simulink model "main"  (R2022a)
settings: Solver=FixedStepDiscrete  StartTime=0.0  StopTime=Inf  FixedStep=(50e-6)-(sim_en*4.995e-5)  RelTol=1e-3  EnableMultiTasking=on
model workspace (MAT data in the model file):
  Param : Simulink.Parameter (value not decoded)
  ac_ok : Simulink.Signal (value not decoded)
  ac_ok_120 : Simulink.Signal (value not decoded)
  bulk_voltage : Simulink.Signal (value not decoded)
  burstduty_integ_max : Simulink.Signal (value not decoded)
  burstduty_integ_min : Simulink.Signal (value not decoded)
  burstduty_ki : Simulink.Signal (value not decoded)
  burstduty_kp : Simulink.Signal (value not decoded)
  calib_ok : Simulink.Signal (value not decoded)
  can_addr1 : Simulink.Signal (value not decoded)
  can_addr2 : Simulink.Signal (value not decoded)
  can_addr3 : Simulink.Signal (value not decoded)
  can_addr4 : Simulink.Signal (value not decoded)
  can_data_rx : Simulink.Signal (value not decoded)
  can_data_tx : Simulink.Signal (value not decoded)
  can_timeout_120 : Simulink.Signal (value not decoded)
  chksum_scircv : Simulink.Signal (value not decoded)
  clllc_en_120 : Simulink.Signal (value not decoded)
  clllc_fault_120 : Simulink.Signal (value not decoded)
  clllc_ok_120 : Simulink.Signal (value not decoded)
  cmpss1h : Simulink.Signal (value not decoded)
  cmpss1l : Simulink.Signal (value not decoded)
  cmpss2h : Simulink.Signal (value not decoded)
  cmpss2l : Simulink.Signal (value not decoded)
  cmpss3h : Simulink.Signal (value not decoded)
  cmpss3l : Simulink.Signal (value not decoded)
  cmpss4h : Simulink.Signal (value not decoded)
  cmpss4l : Simulink.Signal (value not decoded)
  cmpss5h : Simulink.Signal (value not decoded)
  cmpss5l : Simulink.Signal (value not decoded)
  cmpss6h : Simulink.Signal (value not decoded)
  cmpss6l : Simulink.Signal (value not decoded)
  cmpss7h : Simulink.Signal (value not decoded)
  cmpss7l : Simulink.Signal (value not decoded)
  cmpss8h : Simulink.Signal (value not decoded)
  cmpss8l : Simulink.Signal (value not decoded)
  cnt_idle : Simulink.Signal (value not decoded)
  cnt_orps : Simulink.Signal (value not decoded)
  cnt_scircv : Simulink.Signal (value not decoded)
  cnt_scixmt : Simulink.Signal (value not decoded)
  cnt_scixmt_func : Simulink.Signal (value not decoded)
  cnt_temp_mux : Simulink.Signal (value not decoded)
  cnt_vdroop : Simulink.Signal (value not decoded)
  config_ok : Simulink.Signal (value not decoded)
  control_en : Simulink.Signal (value not decoded)
  cp_ready_120 : Simulink.Signal (value not decoded)
  d2d_en : Simulink.Signal (value not decoded)
  dchg_off : Simulink.Signal (value not decoded)
  debug_dacb : Simulink.Signal (value not decoded)
  debug_dacc : Simulink.Signal (value not decoded)
  debug_msg1 : Simulink.Signal (value not decoded)
  debug_msg2 : Simulink.Signal (value not decoded)
  debug_msg3 : Simulink.Signal (value not decoded)
  debug_msg4 : Simulink.Signal (value not decoded)
  debug_msg5 : Simulink.Signal (value not decoded)
  debug_msg6 : Simulink.Signal (value not decoded)
  dir_v2g : Simulink.Signal (value not decoded)
  eoss_llc1 : Simulink.Signal (value not decoded)
  eoss_llc2 : Simulink.Signal (value not decoded)
  eoss_orps : Simulink.Signal (value not decoded)
  fault_ocp : Simulink.Signal (value not decoded)
  fault_otp : Simulink.Signal (value not decoded)
  fault_ovp : Simulink.Signal (value not decoded)
  fut_en : Simulink.Signal (value not decoded)
  fwd_en_120 : Simulink.Signal (value not decoded)
  gain_llc1_sec_idc : Simulink.Signal (value not decoded)
  gain_llc1_temp_sr : Simulink.Signal (value not decoded)
  gain_llc2_sec_idc : Simulink.Signal (value not decoded)
  gain_vbat : Simulink.Signal (value not decoded)
  gain_vbulk : Simulink.Signal (value not decoded)
  gain_vout : Simulink.Signal (value not decoded)
  input_current_phasea : Simulink.Signal (value not decoded)
  input_current_phaseb : Simulink.Signal (value not decoded)
  input_current_phasec : Simulink.Signal (value not decoded)
  input_freq : Simulink.Signal (value not decoded)
  input_power : Simulink.Signal (value not decoded)
  input_voltage_phasea : Simulink.Signal (value not decoded)
  input_voltage_phaseb : Simulink.Signal (value not decoded)
  input_voltage_phasec : Simulink.Signal (value not decoded)
  ishare_arbiter : Simulink.Signal (value not decoded)
  ishare_thresh : Simulink.Signal (value not decoded)
  led_g : Simulink.Signal (value not decoded)
  led_r : Simulink.Signal (value not decoded)
  led_y : Simulink.Signal (value not decoded)
  llc1_burst_integ : Simulink.Signal (value not decoded)
  llc1_burstduty_buffer : Simulink.Signal (value not decoded)
  llc1_pfm_error : Simulink.Signal (value not decoded)
  llc1_pfm_integ : Simulink.Signal (value not decoded)
  llc1_pfm_prop : Simulink.Signal (value not decoded)
  llc1_pri_idc : Simulink.Signal (value not decoded)
  llc1_ps_buffer : Simulink.Signal (value not decoded)
  llc1_pspwm_error : Simulink.Signal (value not decoded)
  llc1_pspwm_integ : Simulink.Signal (value not decoded)
  llc1_pspwm_prop : Simulink.Signal (value not decoded)
  llc1_sec_idc : Simulink.Signal (value not decoded)
  llc1_temp_sr : Simulink.Signal (value not decoded)
  llc1_ts_tbctr_buffer : Simulink.Signal (value not decoded)
  llc2_burst_integ : Simulink.Signal (value not decoded)
  llc2_burstduty_buffer : Simulink.Signal (value not decoded)
  llc2_en : Simulink.Signal (value not decoded)
  llc2_en_buffer : Simulink.Signal (value not decoded)
  llc2_pfm_error : Simulink.Signal (value not decoded)
  llc2_pfm_integ : Simulink.Signal (value not decoded)
  llc2_pfm_prop : Simulink.Signal (value not decoded)
  llc2_pri_idc : Simulink.Signal (value not decoded)
  llc2_ps_buffer : Simulink.Signal (value not decoded)
  llc2_pspwm_error : Simulink.Signal (value not decoded)
  llc2_pspwm_integ : Simulink.Signal (value not decoded)
  llc2_pspwm_prop : Simulink.Signal (value not decoded)
  llc2_sec_idc : Simulink.Signal (value not decoded)
  llc2_temp_sr : Simulink.Signal (value not decoded)
  llc2_ts_tbctr_buffer : Simulink.Signal (value not decoded)
  loop_adcint : Simulink.Signal (value not decoded)
  loop_control : Simulink.Signal (value not decoded)
  loop_idle : Simulink.Signal (value not decoded)
  mid_bulk_voltage : Simulink.Signal (value not decoded)
  mode_120 : Simulink.Signal (value not decoded)
  mode_cc_cv : Simulink.Signal (value not decoded)
  myParam : mpt.Parameter (value not decoded)
  obc_ok_120 : Simulink.Signal (value not decoded)
  offset_llc1_sec_idc : Simulink.Signal (value not decoded)
  offset_llc1_temp_sr : Simulink.Signal (value not decoded)
  offset_llc2_sec_idc : Simulink.Signal (value not decoded)
  offset_vbat : Simulink.Signal (value not decoded)
  offset_vbulk : Simulink.Signal (value not decoded)
  offset_vout : Simulink.Signal (value not decoded)
  openloop_en : Simulink.Signal (value not decoded)
  openloop_fault_en : Simulink.Signal (value not decoded)
  ot_fault_120 : Simulink.Signal (value not decoded)
  pfc_en : Simulink.Signal (value not decoded)
  pfc_en_120 : Simulink.Signal (value not decoded)
  pfc_fw_revision : Simulink.Signal (value not decoded)
  pfc_fw_revision_bootloader : Simulink.Signal (value not decoded)
  pfc_fw_revision_debug : Simulink.Signal (value not decoded)
  pfc_ok : Simulink.Signal (value not decoded)
  pfc_ok_120 : Simulink.Signal (value not decoded)
  pfm_a0 : Simulink.Signal (value not decoded)
  pfm_a1 : Simulink.Signal (value not decoded)
  pfm_integ_max : Simulink.Signal (value not decoded)
  pfm_integ_min : Simulink.Signal (value not decoded)
  pfm_ki : Simulink.Signal (value not decoded)
  pfm_kp : Simulink.Signal (value not decoded)
  pri_fut_en : Simulink.Signal (value not decoded)
  pri_fut_en_buffer : Simulink.Signal (value not decoded)
  pri_halfbridge_en : Simulink.Signal (value not decoded)
  pri_halfbridge_en_buffer : Simulink.Signal (value not decoded)
  pspwm_integ_max : Simulink.Signal (value not decoded)
  pspwm_integ_min : Simulink.Signal (value not decoded)
  pspwm_ki : Simulink.Signal (value not decoded)
  pspwm_kp : Simulink.Signal (value not decoded)
  ref_idclink_max : Simulink.Signal (value not decoded)
  ref_iout : Simulink.Signal (value not decoded)
  ref_iout_calib : Simulink.Signal (value not decoded)
  ref_iout_llc1 : Simulink.Signal (value not decoded)
  ref_iout_llc1_calib : Simulink.Signal (value not decoded)
  ref_iout_llc2 : Simulink.Signal (value not decoded)
  ref_iout_llc2_calib : Simulink.Signal (value not decoded)
  ref_pout : Simulink.Signal (value not decoded)
  ref_ss_llc1 : Simulink.Signal (value not decoded)
  ref_ss_llc2 : Simulink.Signal (value not decoded)
  ref_ss_orps : Simulink.Signal (value not decoded)
  ref_vbat : Simulink.Signal (value not decoded)
  ref_vbat_calib : Simulink.Signal (value not decoded)
  ref_vbulk : Simulink.Signal (value not decoded)
  ref_vbulk_calib : Simulink.Signal (value not decoded)
  ref_vbulk_llc1_calib : Simulink.Signal (value not decoded)
  ref_vbulk_llc2_calib : Simulink.Signal (value not decoded)
  ref_vout : Simulink.Signal (value not decoded)
  ref_vout_calib : Simulink.Signal (value not decoded)
  relay_en : Simulink.Signal (value not decoded)
  reset_flag : Simulink.Signal (value not decoded)
  rev_en_120 : Simulink.Signal (value not decoded)
  runtime_control : Simulink.Signal (value not decoded)
  runtime_idle : Simulink.Signal (value not decoded)
  scircv_buffer : Simulink.Signal (value not decoded)
  scircv_buffer_tmp : Simulink.Signal (value not decoded)
  scircv_buffer_tmp_idx0 : Simulink.Signal (value not decoded)
  scircv_chksum : Simulink.Signal (value not decoded)
  scircv_chksum_ok : Simulink.Signal (value not decoded)
  scircv_parse_ok : Simulink.Signal (value not decoded)
  scixmt_buffer : Simulink.Signal (value not decoded)
  scixmt_chksum : Simulink.Signal (value not decoded)
  scixmt_func : Simulink.Signal (value not decoded)
  scixmt_word0_lsb : Simulink.Signal (value not decoded)
  scixmt_word0_msb : Simulink.Signal (value not decoded)
  scixmt_word1_lsb : Simulink.Signal (value not decoded)
  scixmt_word1_msb : Simulink.Signal (value not decoded)
  scixmt_word2_lsb : Simulink.Signal (value not decoded)
  scixmt_word2_msb : Simulink.Signal (value not decoded)
  scixmt_wr : Simulink.Signal (value not decoded)
  ss_step : Simulink.Signal (value not decoded)
  state_calib : Simulink.Signal (value not decoded)
  state_control : Simulink.Signal (value not decoded)
  state_hkeep : Simulink.Signal (value not decoded)
  status_cmpss : Simulink.Signal (value not decoded)
  status_control : Simulink.Signal (value not decoded)
  status_digin : Simulink.Signal (value not decoded)
  status_digout : Simulink.Signal (value not decoded)
  status_fault : Simulink.Signal (value not decoded)
  status_input : Simulink.Signal (value not decoded)
  status_pfc : Simulink.Signal (value not decoded)
  temp_inlet : Simulink.Signal (value not decoded)
  temp_llc1_fet_hs : Simulink.Signal (value not decoded)
  temp_llc2_fet_hs : Simulink.Signal (value not decoded)
  temp_mux : Simulink.Signal (value not decoded)
  temp_mux_s0 : Simulink.Signal (value not decoded)
  temp_mux_s1 : Simulink.Signal (value not decoded)
  temp_mux_s2 : Simulink.Signal (value not decoded)
  temp_outlet : Simulink.Signal (value not decoded)
  temp_pfc_fet_hsa : Simulink.Signal (value not decoded)
  temp_pfc_fet_hsb : Simulink.Signal (value not decoded)
  temp_pfc_fet_hsc : Simulink.Signal (value not decoded)
  temp_pfc_fet_lsa : Simulink.Signal (value not decoded)
  temp_pfc_fet_lsb : Simulink.Signal (value not decoded)
  temp_pfc_fet_lsc : Simulink.Signal (value not decoded)
  test_mode : Simulink.Signal (value not decoded)
  tfcv_cc : Simulink.Signal (value not decoded)
  tfcv_cc_llc2 : Simulink.Signal (value not decoded)
  tfcv_cv : Simulink.Signal (value not decoded)
  tfcv_sr_en : Simulink.Signal (value not decoded)
  tfv_assert_llc1_pri_idc : Simulink.Signal (value not decoded)
  tfv_assert_llc1_sec_idc : Simulink.Signal (value not decoded)
  tfv_assert_llc1_temp_sr : Simulink.Signal (value not decoded)
  tfv_assert_llc2_pri_idc : Simulink.Signal (value not decoded)
  tfv_assert_llc2_sec_idc : Simulink.Signal (value not decoded)
  tfv_assert_llc2_temp_sr : Simulink.Signal (value not decoded)
  tfv_assert_temp_outlet : Simulink.Signal (value not decoded)
  tfv_assert_vaux_uv : Simulink.Signal (value not decoded)
  tfv_assert_vbat : Simulink.Signal (value not decoded)
  tfv_assert_vbulk : Simulink.Signal (value not decoded)
  tfv_assert_vout : Simulink.Signal (value not decoded)
  tfv_cnt_tz : Simulink.Signal (value not decoded)
  tfv_deassert_llc1_pri_idc : Simulink.Signal (value not decoded)
  tfv_deassert_llc1_sec_idc : Simulink.Signal (value not decoded)
  tfv_deassert_llc1_temp_sr : Simulink.Signal (value not decoded)
  tfv_deassert_llc2_pri_idc : Simulink.Signal (value not decoded)
  tfv_deassert_llc2_sec_idc : Simulink.Signal (value not decoded)
  tfv_deassert_llc2_temp_sr : Simulink.Signal (value not decoded)
  tfv_deassert_temp_outlet : Simulink.Signal (value not decoded)
  tfv_deassert_vaux_uv : Simulink.Signal (value not decoded)
  tfv_deassert_vbat : Simulink.Signal (value not decoded)
  tfv_deassert_vbulk : Simulink.Signal (value not decoded)
  tfv_deassert_vout : Simulink.Signal (value not decoded)
  tfv_llc1_pri_idc : Simulink.Signal (value not decoded)
  tfv_llc1_sec_idc : Simulink.Signal (value not decoded)
  tfv_llc1_temp_sr : Simulink.Signal (value not decoded)
  tfv_llc2_pri_idc : Simulink.Signal (value not decoded)
  tfv_llc2_sec_idc : Simulink.Signal (value not decoded)
  tfv_llc2_temp_sr : Simulink.Signal (value not decoded)
  tfv_temp_outlet : Simulink.Signal (value not decoded)
  tfv_vaux_uv : Simulink.Signal (value not decoded)
  tfv_vbat : Simulink.Signal (value not decoded)
  tfv_vbulk : Simulink.Signal (value not decoded)
  tfv_vout : Simulink.Signal (value not decoded)
  timer_1ms : Simulink.Signal (value not decoded)
  tz : Simulink.Signal (value not decoded)
  valve_en : Simulink.Signal (value not decoded)
  vaux : Simulink.Signal (value not decoded)
  vbat : Simulink.Signal (value not decoded)
  vbulk : Simulink.Signal (value not decoded)
  vout : Simulink.Signal (value not decoded)
undefined symbols (not defined in the file or in its folder): CAN_O_INT, CANA_BASE, Down, GPTRIP1SEL, GPTRIP2SEL, TZ1, TZ2, Up
libraries: hdlsllib x159, simulink x94, c2802xlib x32, c2837xDlib x19, c2807xlib x16, c280xlib x13, canmsglib x8, idelinklib_common x2, c2000lib x1, c281xlib x1
(part 8 of 20)

== system main/Task_Manager/Tmr_1mS/codegen ==
  Task_1mS : Subsystem  TreatAsAtomicUnit=on  ScheduleAs=Periodic partition  PartitionName=Task1mS  SystemSampleTime=1e-3
      settings: RTWFcnNameOpts=Use subsystem name  RTWFileNameOpts=Use subsystem name

== system main/Task_Manager/Tmr_1mS/sim ==

== system main/Task_Manager/Tmr_1s/codegen ==
  Task_1S : Subsystem  TreatAsAtomicUnit=on  ScheduleAs=Periodic partition  PartitionName=Task1S  SystemSampleTime=1
      settings: RTWFcnNameOpts=Use subsystem name  RTWFileNameOpts=Use subsystem name

== system main/Task_Manager/Tmr_1s/sim ==

== system main/Task_Manager/Tmr_20mS/codegen ==
  Task_20mS : Subsystem  TreatAsAtomicUnit=on  ScheduleAs=Periodic partition  PartitionName=Task20mS  SystemSampleTime=19e-3
      settings: RTWFcnNameOpts=Use subsystem name  RTWFileNameOpts=Use subsystem name

== system main/Task_Manager/Tmr_20mS/sim ==

== system main/Task_Manager/idle/cnt_idle ==
  function : TriggerPort  TriggerType=function-call  VariantControl=Variant
  Data Store Read : DataStoreRead  DataStoreName=cnt_idle  IndexOptions=Index vector (dialog)  Indices=1  OutputSizes=1
  If : If  IfExpression=u1 < 5
  cnt_idle : Subsystem  TreatAsAtomicUnit=on
  cnt_idle_sat : Subsystem  TreatAsAtomicUnit=on
  wires:
  Data Store Read/1 -> If/1
  If/1 -> cnt_idle/Action
  If/2 -> cnt_idle_sat/Action

== system main/Task_Manager/idle/idle_task ==
  sim_digin : Inport
  function : TriggerPort  TriggerType=function-call  VariantControl=Variant
  Data Store Read : DataStoreRead  DataStoreName=cnt_idle  IndexOptions=Index vector (dialog)  Indices=1  OutputSizes=1
  Switch Case : SwitchCase  CaseConditions={0,1,2,3,4,5}
  calib : Subsystem  TreatAsAtomicUnit=on
  comm_npc : Subsystem  Commented=on  TreatAsAtomicUnit=on
  debug_dac : Subsystem  Commented=on  TreatAsAtomicUnit=on
  debug_uart1 : Subsystem  Commented=on  TreatAsAtomicUnit=on
  hkeep : Subsystem  TreatAsAtomicUnit=on
  status : Subsystem  TreatAsAtomicUnit=on
  uartx : Subsystem  Commented=on  TreatAsAtomicUnit=on
  watchdog : Subsystem  TreatAsAtomicUnit=on
  sim_digout : Outport
  wires:
  Switch Case/1 -> watchdog/Action
  Switch Case/3 -> hkeep/Action
  Switch Case/5 -> comm_npc/Action
  Switch Case/6 -> debug_dac/Action
  status/1(sim_digout) -> sim_digout/1
  Switch Case/4 -> status/Action
  Data Store Read/1 -> Switch Case/1
  Switch Case/2 -> calib/Action
  sim_digin/1 -> status/1(sim_digin)

== system main/Task_Manager/init/codegen ==
  init : Subsystem
      settings: RTWSystemCode=Inline  RTWFcnNameOpts=Use subsystem name  RTWFileNameOpts=Use subsystem name

== system main/Task_Manager/init/sim ==

== system main/interrupt_adca/burst_control/burst/disPulse ==
  f : TriggerPort  TriggerType=function-call  VariantControl=(inherit)
      settings: CopyFcn=Stateflow.SLINSF.SimulinkMan.removeBlockPreDeleteFcn  PreDeleteFcn=Stateflow.SLINSF.SimulinkMan.unsafePredeleteFcn
  Data Store Read1 : DataStoreRead  DataStoreName=dir_v2g  IndexOptions=Index vector (dialog)  Indices=1  OutputSizes=1
  Rate Transition : RateTransition  Deterministic=off
  Variant Subsystem : Subsystem  Variant=on
  wires:
  Data Store Read1/1 -> Rate Transition/1
  Rate Transition/1 -> Variant Subsystem/1(dir_v2g)

== system main/interrupt_adca/burst_control/burst/disPwm ==
  f : TriggerPort  TriggerType=function-call  VariantControl=(inherit)
      settings: CopyFcn=Stateflow.SLINSF.SimulinkMan.removeBlockPreDeleteFcn  PreDeleteFcn=Stateflow.SLINSF.SimulinkMan.unsafePredeleteFcn
  disPwm : Subsystem  Variant=on

== system main/interrupt_adca/burst_control/burst/enPulse ==
  f : TriggerPort  TriggerType=function-call  VariantControl=(inherit)
      settings: CopyFcn=Stateflow.SLINSF.SimulinkMan.removeBlockPreDeleteFcn  PreDeleteFcn=Stateflow.SLINSF.SimulinkMan.unsafePredeleteFcn
  enPwm : Subsystem  Variant=on

== system main/interrupt_adca/get_adc/adc_variant_subsystem ==
  note: 1) Add Subsystem or Model blocks as valid variant choices.
      | 2) You cannot connect blocks at this level. At simulation, connectivity is automatically
      | determined, based on the active variant and port name matching.
  note: ADCA:
      | llc1_sec_idc
      | llc1_pri_idc
      | vout
  note: ADCB :
      | vaux
      | vbulk
      | temp_mux
  sim_adca : Inport
  sim_adcb : Inport  Port=2
  codegen : Subsystem  VariantControl=sim_en==0
  sim : Subsystem  VariantControl=sim_en==1

== system main/interrupt_adca/to_simulated_plant/codegen ==
  signal_pwm_cllc1 : Outport

== system main/interrupt_adca/to_simulated_plant/sim ==
  Data Store Read3 : DataStoreRead  DataStoreName=llc1_ps  IndexOptions=Index vector (dialog)  Indices=1  OutputSizes=1
  Data Store Read4 : DataStoreRead  DataStoreName=llc1_ts_tbctr  IndexOptions=Index vector (dialog)  Indices=1  OutputSizes=1
  Mux2 : Mux  Inputs=2
  signal_pwm_cllc1 : Outport
  wires:
  Data Store Read4/1 -> Mux2/1
  Data Store Read3/1 -> Mux2/2
  Mux2/1 -> signal_pwm_cllc1/1

== system main/interrupt_canrx/canrx_variant_subsystem/codegen ==
  Function-Call Generator2 : simulink/Ports & Subsystems/Function-Call Generator  sample_time=-1  numberOfIterations=1  DisallowWideOutput=off
  can_rcv : Subsystem  TreatAsAtomicUnit=on
  wires:
  Function-Call Generator2/1 -> can_rcv/Trigger

== system main/interrupt_canrx/canrx_variant_subsystem/sim ==
  sim_canrx : Inport
  Data Store Write1 : DataStoreWrite  DataStoreName=f32BurstDuty1  IndexOptions=Index vector (dialog)  Indices=1  OutputSizes=1
  Data Store Write2 : DataStoreWrite  DataStoreName=f32PhaseShift1  IndexOptions=Index vector (dialog)  Indices=1  OutputSizes=1
  Data Store Write3 : DataStoreWrite  DataStoreName=u8OpenLoopEn1  IndexOptions=Index vector (dialog)  Indices=1  OutputSizes=1
  Data Store Write5 : DataStoreWrite  DataStoreName=f32FreqPeriod1  IndexOptions=Index vector (dialog)  Indices=1  OutputSizes=1
  Demux : Demux
  wires:
  sim_canrx/1 -> Demux/1
  Demux/2 -> Data Store Write5/1
  Demux/3 -> Data Store Write2/1
  Demux/4 -> Data Store Write1/1
  Demux/1 -> Data Store Write3/1

== system main/Control_State_Machine/control/configSr/configXbarEpwmtrip/codegen ==
  dir_v2g : Inport
  If : If  IfExpression=(u1==0)  ElseIfExpressions=(u1==1)  ShowElse=off
  g2v_prifullbridge : Subsystem  TreatAsAtomicUnit=on
  v2g_prifullbridge : Subsystem  TreatAsAtomicUnit=on
  wires:
  dir_v2g/1 -> If/1
  If/2 -> v2g_prifullbridge/Action
  If/1 -> g2v_prifullbridge/Action

== system main/Control_State_Machine/control/configSr/configXbarEpwmtrip/sim ==
  dir_v2g : Inport
  If : If  IfExpression=(u1==0)
  g2v_prifullbridge : Subsystem  TreatAsAtomicUnit=on
  v2g_prifullbridge : Subsystem  TreatAsAtomicUnit=on
  wires:
  If/2 -> v2g_prifullbridge/Action
  dir_v2g/1 -> If/1
  If/1 -> g2v_prifullbridge/Action

== system main/Control_State_Machine/control/disPwm/disPwm/codegen ==
  note: EPwm1Regs.AQCSFRC.bit.CSFA = 0b01; //force low
      | EPwm1Regs.AQCSFRC.bit.CSFB = 0b01; //force low
      | EPwm2Regs.AQCSFRC.bit.CSFA = 0b01; //force low
      | EPwm2Regs.AQCSFRC.bit.CSFB = 0b01; //force low
      |
      | EPwm7Regs.AQCSFRC.bit.CSFA = 0b01; //force low
      | EPwm7Regs.AQCSFRC.bit.CSFB = 0b01; //force low
      | EPwm8Regs.AQCSFRC.bit.CSFA = 0b01; //force low
      | EPwm8Regs.AQCSFRC.bit.CSFB = 0b01; //force low
  System Outputs1 : Subsystem  VariantControl=Choice  mask(System Outputs){ShowInLibBrowser=0}
      mask prompts: ShowInLibBrowser "Simulink:masks:CustCodeMaskParam1_MP"
      settings: CopyFcn=cccopyfcn(gcb)  OpenFcn=ccopenfcn('System Outputs Function')
      mask Help: eval('feval(''rtwprivate'',''rtwhelpview'',''rtw_sys_outputs_block'')');
      mask DialogControl ShowInLibBrowser Prompt: Mask Parameter 1:
      mask Display: disp('System\nOutputs');

== system main/Control_State_Machine/control/disPwm/disPwm/sim ==
  note: Note:
      | 0 - disable forced low
      | 1 - forced low
  Constant : Constant  OutDataTypeStr=boolean
  Data Store Write : DataStoreWrite  DataStoreName=epwm1_aqcsfrc_csfa  IndexOptions=Index vector (dialog)  Indices=1  OutputSizes=1
  Data Store Write1 : DataStoreWrite  DataStoreName=epwm1_aqcsfrc_csfb  IndexOptions=Index vector (dialog)  Indices=1  OutputSizes=1
  Data Store Write2 : DataStoreWrite  DataStoreName=epwm2_aqcsfrc_csfa  IndexOptions=Index vector (dialog)  Indices=1  OutputSizes=1
  Data Store Write3 : DataStoreWrite  DataStoreName=epwm2_aqcsfrc_csfb  IndexOptions=Index vector (dialog)  Indices=1  OutputSizes=1
  Data Store Write4 : DataStoreWrite  DataStoreName=epwm7_aqcsfrc_csfa  IndexOptions=Index vector (dialog)  Indices=1  OutputSizes=1
  Data Store Write5 : DataStoreWrite  DataStoreName=epwm7_aqcsfrc_csfb  IndexOptions=Index vector (dialog)  Indices=1  OutputSizes=1
  Data Store Write6 : DataStoreWrite  DataStoreName=epwm8_aqcsfrc_csfa  IndexOptions=Index vector (dialog)  Indices=1  OutputSizes=1
  Data Store Write7 : DataStoreWrite  DataStoreName=epwm8_aqcsfrc_csfb  IndexOptions=Index vector (dialog)  Indices=1  OutputSizes=1
  wires:
  Constant/1 -> Data Store Write7/1, Data Store Write6/1, Data Store Write5/1, Data Store Write4/1, Data Store Write3/1, Data Store Write2/1, Data Store Write1/1, Data Store Write/1

== system main/Control_State_Machine/control/enableSR/enPwm/codegen ==
  note: EPwm1Regs.AQCSFRC.bit.CSFA = 0b0; //force disabled
      | EPwm1Regs.AQCSFRC.bit.CSFB = 0b0; //force disabled
      | EPwm2Regs.AQCSFRC.bit.CSFA = 0b0; //force disabled
      | EPwm2Regs.AQCSFRC.bit.CSFB = 0b0; //force disabled
      |
      | //Enable sync  rec
      | //EPwm7Regs.AQCSFRC.bit.CSFA = 0b0; //force disabled
      | //EPwm7Regs.AQCSFRC.bit.CSFB = 0b0; //force disabled
      | //EPwm8Regs.AQCSFRC.bit.CSFA = 0b0; //force disabled
      | //EPwm8Regs.AQCSFRC.bit.CSFB = 0b0; //force disabled
      |
      | //Disable sync rec
      | EPwm7Regs.AQCSFRC.bit.CSFA = 0b1; //force low
      | EPwm7Regs.AQCSFRC.bit.CSFB = 0b1; //force low
      | EPwm8Regs.AQCSFRC.bit.CSFA = 0b1; //force low
      | EPwm8Regs.AQCSFRC.bit.CSFB = 0b1; //force low
  System Outputs : Subsystem  mask(System Outputs){ShowInLibBrowser=0}
      mask prompts: ShowInLibBrowser "Simulink:masks:CustCodeMaskParam1_MP"
      settings: CopyFcn=cccopyfcn(gcb)  OpenFcn=ccopenfcn('System Outputs Function')
      mask Help: eval('feval(''rtwprivate'',''rtwhelpview'',''rtw_sys_outputs_block'')');
      mask Display: disp('System\nOutputs');

== system main/Control_State_Machine/control/enableSR/enPwm/sim ==
  note: LLC1 SEC
  note: LLC1 PRI
  note: EPwm1Regs.AQCSFRC.bit.CSFA = 0b0; //force disabled
      | EPwm1Regs.AQCSFRC.bit.CSFB = 0b0; //force disabled
      | EPwm2Regs.AQCSFRC.bit.CSFA = 0b0; //force disabled
      | EPwm2Regs.AQCSFRC.bit.CSFB = 0b0; //force disabled
      | EPwm7Regs.AQCSFRC.bit.CSFA = 0b0; //force disabled
      | EPwm7Regs.AQCSFRC.bit.CSFB = 0b0; //force disabled
      | EPwm8Regs.AQCSFRC.bit.CSFA = 0b0; //force disabled
      | EPwm8Regs.AQCSFRC.bit.CSFB = 0b0; //force disabled
  Constant{,1..7} (8 alike) : Constant  Value=0  OutDataTypeStr=boolean
  Data Store Write : DataStoreWrite  DataStoreName=epwm1_aqcsfrc_csfa  IndexOptions=Index vector (dialog)  Indices=1  OutputSizes=1
  Data Store Write1 : DataStoreWrite  DataStoreName=epwm1_aqcsfrc_csfb  IndexOptions=Index vector (dialog)  Indices=1  OutputSizes=1
  Data Store Write2 : DataStoreWrite  DataStoreName=epwm7_aqcsfrc_csfa  IndexOptions=Index vector (dialog)  Indices=1  OutputSizes=1
  Data Store Write3 : DataStoreWrite  DataStoreName=epwm7_aqcsfrc_csfb  IndexOptions=Index vector (dialog)  Indices=1  OutputSizes=1
  Data Store Write4 : DataStoreWrite  DataStoreName=epwm2_aqcsfrc_csfa  IndexOptions=Index vector (dialog)  Indices=1  OutputSizes=1
  Data Store Write5 : DataStoreWrite  DataStoreName=epwm2_aqcsfrc_csfb  IndexOptions=Index vector (dialog)  Indices=1  OutputSizes=1
  Data Store Write6 : DataStoreWrite  DataStoreName=epwm8_aqcsfrc_csfa  IndexOptions=Index vector (dialog)  Indices=1  OutputSizes=1
  Data Store Write7 : DataStoreWrite  DataStoreName=epwm8_aqcsfrc_csfb  IndexOptions=Index vector (dialog)  Indices=1  OutputSizes=1
  wires:
  Constant/1 -> Data Store Write/1
  Constant1/1 -> Data Store Write1/1
  Constant4/1 -> Data Store Write4/1
  Constant5/1 -> Data Store Write5/1
  Constant7/1 -> Data Store Write7/1
  Constant6/1 -> Data Store Write6/1
  Constant3/1 -> Data Store Write3/1
  Constant2/1 -> Data Store Write2/1

== system main/Control_State_Machine/control/initG2vCcBurst/initG2vCcBurst/codegen ==
  Constant : Constant  Value=0.0025  OutDataTypeStr=single
  Constant1 : Constant  Value=0.00025  OutDataTypeStr=single
  Constant2 : Constant  Value=0  OutDataTypeStr=single
  Constant3 : Constant  Value=100  OutDataTypeStr=single
  Data Store Write : DataStoreWrite  DataStoreName=burstduty_kp  IndexOptions=Index vector (dialog)  Indices=1  OutputSizes=1
  Data Store Write1 : DataStoreWrite  DataStoreName=burstduty_ki  IndexOptions=Index vector (dialog)  Indices=1  OutputSizes=1
  Data Store Write2 : DataStoreWrite  DataStoreName=burstduty_integ_min  IndexOptions=Index vector (dialog)  Indices=1  OutputSizes=1
  Data Store Write3 : DataStoreWrite  DataStoreName=burstduty_integ_max  IndexOptions=Index vector (dialog)  Indices=1  OutputSizes=1
  wires:
  Constant3/1 -> Data Store Write3/1
  Constant2/1 -> Data Store Write2/1
  Constant1/1 -> Data Store Write1/1
  Constant/1 -> Data Store Write/1

== system main/Control_State_Machine/control/initG2vCcBurst/initG2vCcBurst/sim ==
  Constant : Constant  Value=40e-1  OutDataTypeStr=single
  Constant1 : Constant  Value=40e-2  OutDataTypeStr=single
  Constant2 : Constant  Value=0  OutDataTypeStr=single
  Constant3 : Constant  Value=100  OutDataTypeStr=single
  Data Store Write : DataStoreWrite  DataStoreName=burstduty_kp  IndexOptions=Index vector (dialog)  Indices=1  OutputSizes=1
  Data Store Write1 : DataStoreWrite  DataStoreName=burstduty_ki  IndexOptions=Index vector (dialog)  Indices=1  OutputSizes=1
  Data Store Write2 : DataStoreWrite  DataStoreName=burstduty_integ_min  IndexOptions=Index vector (dialog)  Indices=1  OutputSizes=1
  Data Store Write3 : DataStoreWrite  DataStoreName=burstduty_integ_max  IndexOptions=Index vector (dialog)  Indices=1  OutputSizes=1
  wires:
  Constant2/1 -> Data Store Write2/1
  Constant3/1 -> Data Store Write3/1
  Constant1/1 -> Data Store Write1/1
  Constant/1 -> Data Store Write/1

== system main/Control_State_Machine/control/initG2vCcPfm/initG2vCcPfm/codegen ==
  Constant : Constant  Value=0.041557  OutDataTypeStr=single
  Constant1 : Constant  Value=-0.02169  OutDataTypeStr=single
  Constant2 : Constant  Value=333  OutDataTypeStr=single
  Constant3 : Constant  Value=2000  OutDataTypeStr=single
  Constant4 : Constant  Commented=on  Value=0.2835  OutDataTypeStr=single
  Constant5 : Constant  Commented=on  Value=-0.2188  OutDataTypeStr=single
  Data Store Write4 : DataStoreWrite  DataStoreName=pfm_kp  IndexOptions=Index vector (dialog)  Indices=1  OutputSizes=1
  Data Store Write5 : DataStoreWrite  DataStoreName=pfm_ki  IndexOptions=Index vector (dialog)  Indices=1  OutputSizes=1
  Data Store Write6 : DataStoreWrite  DataStoreName=pfm_integ_min  IndexOptions=Index vector (dialog)  Indices=1  OutputSizes=1
  Data Store Write7 : DataStoreWrite  DataStoreName=pfm_integ_max  IndexOptions=Index vector (dialog)  Indices=1  OutputSizes=1
  wires:
  Constant2/1 -> Data Store Write6/1
  Constant1/1 -> Data Store Write5/1
  Constant3/1 -> Data Store Write7/1
  Constant/1 -> Data Store Write4/1

== system main/Control_State_Machine/control/initG2vCcPfm/initG2vCcPfm/sim ==
  Constant : Constant  Commented=on  Value=2.2e-2  OutDataTypeStr=single
  Constant1 : Constant  Commented=on  Value=2.2e-3  OutDataTypeStr=single
  Constant2 : Constant  Value=333  OutDataTypeStr=single
  Constant3 : Constant  Value=2000  OutDataTypeStr=single
  Constant4 : Constant  Value=0.1314  OutDataTypeStr=single
  Constant5 : Constant  Value=-0.06858  OutDataTypeStr=single
  Data Store Write1 : DataStoreWrite  DataStoreName=pfm_a0  IndexOptions=Index vector (dialog)  Indices=1  OutputSizes=1
  Data Store Write2 : DataStoreWrite  DataStoreName=pfm_a1  IndexOptions=Index vector (dialog)  Indices=1  OutputSizes=1
  Data Store Write4 : DataStoreWrite  Commented=on  DataStoreName=pfm_kp  IndexOptions=Index vector (dialog)  Indices=1  OutputSizes=1
  Data Store Write5 : DataStoreWrite  Commented=on  DataStoreName=pfm_ki  IndexOptions=Index vector (dialog)  Indices=1  OutputSizes=1
  Data Store Write6 : DataStoreWrite  DataStoreName=pfm_integ_min  IndexOptions=Index vector (dialog)  Indices=1  OutputSizes=1
  Data Store Write7 : DataStoreWrite  DataStoreName=pfm_integ_max  IndexOptions=Index vector (dialog)  Indices=1  OutputSizes=1
  wires:
  Constant/1 -> Data Store Write4/1
  Constant1/1 -> Data Store Write5/1
  Constant2/1 -> Data Store Write6/1
  Constant3/1 -> Data Store Write7/1
  Constant4/1 -> Data Store Write1/1
  Constant5/1 -> Data Store Write2/1

== system main/Control_State_Machine/control/initG2vCcPspwm/initG2vCcPfm/codegen ==
  Constant : Constant  Value=-1e-1  OutDataTypeStr=single
  Constant1 : Constant  Value=-1e-3  OutDataTypeStr=single
  Constant2 : Constant  Value=0  OutDataTypeStr=single
  Constant3 : Constant  Value=36  OutDataTypeStr=single
  Data Store Write : DataStoreWrite  DataStoreName=pspwm_kp  IndexOptions=Index vector (dialog)  Indices=1  OutputSizes=1
  Data Store Write1 : DataStoreWrite  DataStoreName=pspwm_ki  IndexOptions=Index vector (dialog)  Indices=1  OutputSizes=1
  Data Store Write2 : DataStoreWrite  DataStoreName=pspwm_integ_min  IndexOptions=Index vector (dialog)  Indices=1  OutputSizes=1
  Data Store Write3 : DataStoreWrite  DataStoreName=pspwm_integ_max  IndexOptions=Index vector (dialog)  Indices=1  OutputSizes=1
  wires:
  Constant3/1 -> Data Store Write3/1
  Constant2/1 -> Data Store Write2/1
  Constant1/1 -> Data Store Write1/1
  Constant/1 -> Data Store Write/1

== system main/Control_State_Machine/control/initG2vCcPspwm/initG2vCcPfm/sim ==
  Constant : Constant  Value=-1e-1  OutDataTypeStr=single
  Constant1 : Constant  Value=-3e-2  OutDataTypeStr=single
  Constant2 : Constant  Value=0  OutDataTypeStr=single
  Constant3 : Constant  Value=36  OutDataTypeStr=single
  Data Store Write : DataStoreWrite  DataStoreName=pspwm_kp  IndexOptions=Index vector (dialog)  Indices=1  OutputSizes=1
  Data Store Write1 : DataStoreWrite  DataStoreName=pspwm_ki  IndexOptions=Index vector (dialog)  Indices=1  OutputSizes=1
  Data Store Write2 : DataStoreWrite  DataStoreName=pspwm_integ_min  IndexOptions=Index vector (dialog)  Indices=1  OutputSizes=1
  Data Store Write3 : DataStoreWrite  DataStoreName=pspwm_integ_max  IndexOptions=Index vector (dialog)  Indices=1  OutputSizes=1
  wires:
  Constant2/1 -> Data Store Write2/1
  Constant3/1 -> Data Store Write3/1
  Constant1/1 -> Data Store Write1/1
  Constant/1 -> Data Store Write/1

== system main/Control_State_Machine/control/initG2vCvBurst/initG2vCvBurst/codegen ==
  Constant : Constant  Value=0.025  OutDataTypeStr=single
  Constant1 : Constant  Value=0.00025  OutDataTypeStr=single
  Constant2 : Constant  Value=0  OutDataTypeStr=single
  Constant3 : Constant  Value=100  OutDataTypeStr=single
  Data Store Write : DataStoreWrite  DataStoreName=burstduty_kp  IndexOptions=Index vector (dialog)  Indices=1  OutputSizes=1
  Data Store Write1 : DataStoreWrite  DataStoreName=burstduty_ki  IndexOptions=Index vector (dialog)  Indices=1  OutputSizes=1
  Data Store Write2 : DataStoreWrite  DataStoreName=burstduty_integ_min  IndexOptions=Index vector (dialog)  Indices=1  OutputSizes=1
  Data Store Write3 : DataStoreWrite  DataStoreName=burstduty_integ_max  IndexOptions=Index vector (dialog)  Indices=1  OutputSizes=1
  wires:
  Constant3/1 -> Data Store Write3/1
  Constant2/1 -> Data Store Write2/1
  Constant1/1 -> Data Store Write1/1
  Constant/1 -> Data Store Write/1

== system main/Control_State_Machine/control/initG2vCvBurst/initG2vCvBurst/sim ==
  Constant : Constant  Value=40e-1  OutDataTypeStr=single
  Constant1 : Constant  Value=40e-2  OutDataTypeStr=single
  Constant2 : Constant  Value=0  OutDataTypeStr=single
  Constant3 : Constant  Value=100  OutDataTypeStr=single
  Data Store Write : DataStoreWrite  DataStoreName=burstduty_kp  IndexOptions=Index vector (dialog)  Indices=1  OutputSizes=1
  Data Store Write1 : DataStoreWrite  DataStoreName=burstduty_ki  IndexOptions=Index vector (dialog)  Indices=1  OutputSizes=1
  Data Store Write2 : DataStoreWrite  DataStoreName=burstduty_integ_min  IndexOptions=Index vector (dialog)  Indices=1  OutputSizes=1
  Data Store Write3 : DataStoreWrite  DataStoreName=burstduty_integ_max  IndexOptions=Index vector (dialog)  Indices=1  OutputSizes=1
  wires:
  Constant2/1 -> Data Store Write2/1
  Constant3/1 -> Data Store Write3/1
  Constant1/1 -> Data Store Write1/1
  Constant/1 -> Data Store Write/1

== system main/Control_State_Machine/control/initG2vCvPfm/initG2vCvPfm/codegen ==
  Constant : Constant  Value=0.001471  OutDataTypeStr=single
  Constant1 : Constant  Value=-0.000529  OutDataTypeStr=single
  Constant2 : Constant  Value=333  OutDataTypeStr=single
  Constant3 : Constant  Value=2000  OutDataTypeStr=single
  Constant4 : Constant  Commented=on  Value=0.2835  OutDataTypeStr=single
  Constant5 : Constant  Commented=on  Value=-0.2188  OutDataTypeStr=single
  Data Store Write4 : DataStoreWrite  DataStoreName=pfm_kp  IndexOptions=Index vector (dialog)  Indices=1  OutputSizes=1
  Data Store Write5 : DataStoreWrite  DataStoreName=pfm_ki  IndexOptions=Index vector (dialog)  Indices=1  OutputSizes=1
  Data Store Write6 : DataStoreWrite  DataStoreName=pfm_integ_min  IndexOptions=Index vector (dialog)  Indices=1  OutputSizes=1
  Data Store Write7 : DataStoreWrite  DataStoreName=pfm_integ_max  IndexOptions=Index vector (dialog)  Indices=1  OutputSizes=1
  wires:
  Constant2/1 -> Data Store Write6/1
  Constant1/1 -> Data Store Write5/1
  Constant3/1 -> Data Store Write7/1
  Constant/1 -> Data Store Write4/1

== system main/Control_State_Machine/control/initG2vCvPfm/initG2vCvPfm/sim ==
  Constant : Constant  Commented=on  Value=2.2e-2  OutDataTypeStr=single
  Constant1 : Constant  Commented=on  Value=2.2e-3  OutDataTypeStr=single
  Constant2 : Constant  Value=333  OutDataTypeStr=single
  Constant3 : Constant  Value=2000  OutDataTypeStr=single
  Constant4 : Constant  Value=0.1314  OutDataTypeStr=single
  Constant5 : Constant  Value=-0.06858  OutDataTypeStr=single
  Data Store Write1 : DataStoreWrite  DataStoreName=pfm_a0  IndexOptions=Index vector (dialog)  Indices=1  OutputSizes=1
  Data Store Write2 : DataStoreWrite  DataStoreName=pfm_a1  IndexOptions=Index vector (dialog)  Indices=1  OutputSizes=1
  Data Store Write4 : DataStoreWrite  Commented=on  DataStoreName=pfm_kp  IndexOptions=Index vector (dialog)  Indices=1  OutputSizes=1
  Data Store Write5 : DataStoreWrite  Commented=on  DataStoreName=pfm_ki  IndexOptions=Index vector (dialog)  Indices=1  OutputSizes=1
  Data Store Write6 : DataStoreWrite  DataStoreName=pfm_integ_min  IndexOptions=Index vector (dialog)  Indices=1  OutputSizes=1
  Data Store Write7 : DataStoreWrite  DataStoreName=pfm_integ_max  IndexOptions=Index vector (dialog)  Indices=1  OutputSizes=1
  wires:
  Constant/1 -> Data Store Write4/1
  Constant1/1 -> Data Store Write5/1
  Constant2/1 -> Data Store Write6/1
  Constant3/1 -> Data Store Write7/1
  Constant4/1 -> Data Store Write1/1
  Constant5/1 -> Data Store Write2/1

== system main/Control_State_Machine/control/initG2vCvPspwm/initG2vCvPfm/codegen ==
  Constant : Constant  Value=-1e-1  OutDataTypeStr=single
  Constant1 : Constant  Value=-1e-3  OutDataTypeStr=single
  Constant2 : Constant  Value=0  OutDataTypeStr=single
  Constant3 : Constant  Value=36  OutDataTypeStr=single
  Data Store Write : DataStoreWrite  DataStoreName=pspwm_kp  IndexOptions=Index vector (dialog)  Indices=1  OutputSizes=1
  Data Store Write1 : DataStoreWrite  DataStoreName=pspwm_ki  IndexOptions=Index vector (dialog)  Indices=1  OutputSizes=1
  Data Store Write2 : DataStoreWrite  DataStoreName=pspwm_integ_min  IndexOptions=Index vector (dialog)  Indices=1  OutputSizes=1
  Data Store Write3 : DataStoreWrite  DataStoreName=pspwm_integ_max  IndexOptions=Index vector (dialog)  Indices=1  OutputSizes=1
  wires:
  Constant3/1 -> Data Store Write3/1
  Constant2/1 -> Data Store Write2/1
  Constant1/1 -> Data Store Write1/1
  Constant/1 -> Data Store Write/1

== system main/Control_State_Machine/control/initG2vCvPspwm/initG2vCvPfm/sim ==
  Constant : Constant  Value=-1e-1  OutDataTypeStr=single
  Constant1 : Constant  Value=-3e-2  OutDataTypeStr=single
  Constant2 : Constant  Value=0  OutDataTypeStr=single
  Constant3 : Constant  Value=36  OutDataTypeStr=single
  Data Store Write : DataStoreWrite  DataStoreName=pspwm_kp  IndexOptions=Index vector (dialog)  Indices=1  OutputSizes=1
  Data Store Write1 : DataStoreWrite  DataStoreName=pspwm_ki  IndexOptions=Index vector (dialog)  Indices=1  OutputSizes=1
  Data Store Write2 : DataStoreWrite  DataStoreName=pspwm_integ_min  IndexOptions=Index vector (dialog)  Indices=1  OutputSizes=1
  Data Store Write3 : DataStoreWrite  DataStoreName=pspwm_integ_max  IndexOptions=Index vector (dialog)  Indices=1  OutputSizes=1
  wires:
  Constant2/1 -> Data Store Write2/1
  Constant3/1 -> Data Store Write3/1
  Constant1/1 -> Data Store Write1/1
  Constant/1 -> Data Store Write/1

== system main/Control_State_Machine/control/initV2gCvBurst/initV2gCvBurst/codegen ==
  Constant : Constant  Value=0.025  OutDataTypeStr=single
  Constant1 : Constant  Value=0.00025  OutDataTypeStr=single
  Constant2 : Constant  Value=0  OutDataTypeStr=single
  Constant3 : Constant  Value=100  OutDataTypeStr=single
  Data Store Write : DataStoreWrite  DataStoreName=burstduty_kp  IndexOptions=Index vector (dialog)  Indices=1  OutputSizes=1
  Data Store Write1 : DataStoreWrite  DataStoreName=burstduty_ki  IndexOptions=Index vector (dialog)  Indices=1  OutputSizes=1
  Data Store Write2 : DataStoreWrite  DataStoreName=burstduty_integ_min  IndexOptions=Index vector (dialog)  Indices=1  OutputSizes=1
  Data Store Write3 : DataStoreWrite  DataStoreName=burstduty_integ_max  IndexOptions=Index vector (dialog)  Indices=1  OutputSizes=1
  wires:
  Constant3/1 -> Data Store Write3/1
  Constant2/1 -> Data Store Write2/1
  Constant1/1 -> Data Store Write1/1
  Constant/1 -> Data Store Write/1

== system main/Control_State_Machine/control/initV2gCvBurst/initV2gCvBurst/sim ==
  Constant : Constant  Value=8e-1  OutDataTypeStr=single
  Constant1 : Constant  Value=8e-2  OutDataTypeStr=single
  Constant2 : Constant  Value=0  OutDataTypeStr=single
  Constant3 : Constant  Value=100  OutDataTypeStr=single
  Data Store Write : DataStoreWrite  DataStoreName=burstduty_kp  IndexOptions=Index vector (dialog)  Indices=1  OutputSizes=1
  Data Store Write1 : DataStoreWrite  DataStoreName=burstduty_ki  IndexOptions=Index vector (dialog)  Indices=1  OutputSizes=1
  Data Store Write2 : DataStoreWrite  DataStoreName=burstduty_integ_min  IndexOptions=Index vector (dialog)  Indices=1  OutputSizes=1
  Data Store Write3 : DataStoreWrite  DataStoreName=burstduty_integ_max  IndexOptions=Index vector (dialog)  Indices=1  OutputSizes=1
  wires:
  Constant2/1 -> Data Store Write2/1
  Constant3/1 -> Data Store Write3/1
  Constant1/1 -> Data Store Write1/1
  Constant/1 -> Data Store Write/1

== system main/Control_State_Machine/control/initV2gCvPfm/initV2gCvPfm/codegen ==
  Constant : Constant  Value=1e-1  OutDataTypeStr=single
  Constant1 : Constant  Value=1e-5  OutDataTypeStr=single
  Constant2 : Constant  Value=333  OutDataTypeStr=single
  Constant3 : Constant  Value=2000  OutDataTypeStr=single
  Data Store Write4 : DataStoreWrite  DataStoreName=pfm_kp  IndexOptions=Index vector (dialog)  Indices=1  OutputSizes=1
  Data Store Write5 : DataStoreWrite  DataStoreName=pfm_ki  IndexOptions=Index vector (dialog)  Indices=1  OutputSizes=1
  Data Store Write6 : DataStoreWrite  DataStoreName=pfm_integ_min  IndexOptions=Index vector (dialog)  Indices=1  OutputSizes=1
  Data Store Write7 : DataStoreWrite  DataStoreName=pfm_integ_max  IndexOptions=Index vector (dialog)  Indices=1  OutputSizes=1
  wires:
  Constant2/1 -> Data Store Write6/1
  Constant1/1 -> Data Store Write5/1
  Constant3/1 -> Data Store Write7/1
  Constant/1 -> Data Store Write4/1

== system main/Control_State_Machine/control/initV2gCvPfm/initV2gCvPfm/sim ==
  Constant : Constant  Commented=on  Value=0.02381  OutDataTypeStr=single
  Constant1 : Constant  Commented=on  Value=952  OutDataTypeStr=single
  Constant2 : Constant  Value=333  OutDataTypeStr=single
  Constant3 : Constant  Value=2000  OutDataTypeStr=single
  Constant4 : Constant  Value=0.1708  OutDataTypeStr=single
  Constant5 : Constant  Value=-0.1697  OutDataTypeStr=single
  Data Store Write1 : DataStoreWrite  DataStoreName=pfm_a0  IndexOptions=Index vector (dialog)  Indices=1  OutputSizes=1
  Data Store Write2 : DataStoreWrite  DataStoreName=pfm_a1  IndexOptions=Index vector (dialog)  Indices=1  OutputSizes=1
  Data Store Write4 : DataStoreWrite  Commented=on  DataStoreName=pfm_kp  IndexOptions=Index vector (dialog)  Indices=1  OutputSizes=1
  Data Store Write5 : DataStoreWrite  Commented=on  DataStoreName=pfm_ki  IndexOptions=Index vector (dialog)  Indices=1  OutputSizes=1
  Data Store Write6 : DataStoreWrite  DataStoreName=pfm_integ_min  IndexOptions=Index vector (dialog)  Indices=1  OutputSizes=1
  Data Store Write7 : DataStoreWrite  DataStoreName=pfm_integ_max  IndexOptions=Index vector (dialog)  Indices=1  OutputSizes=1
  wires:
  Constant/1 -> Data Store Write4/1
  Constant1/1 -> Data Store Write5/1
  Constant2/1 -> Data Store Write6/1
  Constant3/1 -> Data Store Write7/1
  Constant5/1 -> Data Store Write2/1
  Constant4/1 -> Data Store Write1/1

== system main/Control_State_Machine/control/initV2gCvPspwm/initV2gCvPspwm/codegen ==
  Constant : Constant  Value=-1e-1  OutDataTypeStr=single
  Constant1 : Constant  Value=-1e-3  OutDataTypeStr=single
  Constant2 : Constant  Value=0  OutDataTypeStr=single
  Constant3 : Constant  Value=36  OutDataTypeStr=single
  Data Store Write : DataStoreWrite  DataStoreName=pspwm_kp  IndexOptions=Index vector (dialog)  Indices=1  OutputSizes=1
  Data Store Write1 : DataStoreWrite  DataStoreName=pspwm_ki  IndexOptions=Index vector (dialog)  Indices=1  OutputSizes=1
  Data Store Write2 : DataStoreWrite  DataStoreName=pspwm_integ_min  IndexOptions=Index vector (dialog)  Indices=1  OutputSizes=1
  Data Store Write3 : DataStoreWrite  DataStoreName=pspwm_integ_max  IndexOptions=Index vector (dialog)  Indices=1  OutputSizes=1
  wires:
  Constant3/1 -> Data Store Write3/1
  Constant2/1 -> Data Store Write2/1
  Constant1/1 -> Data Store Write1/1
  Constant/1 -> Data Store Write/1

== system main/Control_State_Machine/control/initV2gCvPspwm/initV2gCvPspwm/sim ==
  Constant : Constant  Value=-6e-1  OutDataTypeStr=single
  Constant1 : Constant  Value=-6e-2  OutDataTypeStr=single
  Constant2 : Constant  Value=0  OutDataTypeStr=single
  Constant3 : Constant  Value=36  OutDataTypeStr=single
  Data Store Write : DataStoreWrite  DataStoreName=pspwm_kp  IndexOptions=Index vector (dialog)  Indices=1  OutputSizes=1
  Data Store Write1 : DataStoreWrite  DataStoreName=pspwm_ki  IndexOptions=Index vector (dialog)  Indices=1  OutputSizes=1
  Data Store Write2 : DataStoreWrite  DataStoreName=pspwm_integ_min  IndexOptions=Index vector (dialog)  Indices=1  OutputSizes=1
  Data Store Write3 : DataStoreWrite  DataStoreName=pspwm_integ_max  IndexOptions=Index vector (dialog)  Indices=1  OutputSizes=1
  wires:
  Constant2/1 -> Data Store Write2/1
  Constant3/1 -> Data Store Write3/1
  Constant1/1 -> Data Store Write1/1
  Constant/1 -> Data Store Write/1

== system main/Task_Manager/Tmr_1mS/codegen/Task_1mS ==
  Counter_1mS : Subsystem  TreatAsAtomicUnit=on
      settings: RTWSystemCode=Inline
  Function-Call Generator1 : simulink/Ports & Subsystems/Function-Call Generator  sample_time=-1  numberOfIterations=1  DisallowWideOutput=off
  Function-Call Split3 : FunctionCallSplit  NumOutputPorts=2
  GPIO_Handler : Subsystem  TreatAsAtomicUnit=on
      settings: RTWSystemCode=Inline
  wires:
  Function-Call Generator1/1 -> Function-Call Split3/1
  Function-Call Split3/1 -> Counter_1mS/Trigger
  Function-Call Split3/2 -> GPIO_Handler/Trigger

== system main/Task_Manager/Tmr_1s/codegen/Task_1S ==
  Function-Call Generator1 : simulink/Ports & Subsystems/Function-Call Generator  sample_time=-1  numberOfIterations=1  DisallowWideOutput=off
  Function-Call Split3 : FunctionCallSplit  NumOutputPorts=2
  addressing_temp_mux : Subsystem  TreatAsAtomicUnit=on
      settings: RTWSystemCode=Inline
  cnt_temp_mux : Subsystem  TreatAsAtomicUnit=on
      settings: RTWSystemCode=Inline
  wires:
  Function-Call Split3/2 -> addressing_temp_mux/Trigger
  Function-Call Split3/1 -> cnt_temp_mux/Trigger
  Function-Call Generator1/1 -> Function-Call Split3/1

== system main/Task_Manager/Tmr_20mS/codegen/Task_20mS ==
  Function-Call Generator1 : simulink/Ports & Subsystems/Function-Call Generator  sample_time=-1  numberOfIterations=1  DisallowWideOutput=off
  Function-Call Split1 : FunctionCallSplit  NumOutputPorts=2
  Rx_Handler : Subsystem  TreatAsAtomicUnit=on
  Tx_Handler : Subsystem  TreatAsAtomicUnit=on
  wires:
  Function-Call Split1/2 -> Tx_Handler/Trigger
  Function-Call Split1/1 -> Rx_Handler/Trigger
  Function-Call Generator1/1 -> Function-Call Split1/1

== system main/Task_Manager/idle/cnt_idle/cnt_idle ==
  Action Port : ActionPort  ActionPortLabel=if(u1 < 5)
  Add : Sum
  Constant : Constant  OutDataTypeStr=uint16
  Data Store Read1 : DataStoreRead  DataStoreName=cnt_idle  IndexOptions=Index vector (dialog)  Indices=1  OutputSizes=1
  Data Store Write : DataStoreWrite  DataStoreName=cnt_idle  IndexOptions=Index vector (dialog)  Indices=1  OutputSizes=1
  wires:
  Data Store Read1/1 -> Add/1
  Add/1 -> Data Store Write/1
  Constant/1 -> Add/2

== system main/Task_Manager/idle/cnt_idle/cnt_idle_sat ==
  Action Port : ActionPort  ActionPortLabel=else
  Constant : Constant  Value=0  OutDataTypeStr=uint16
  Data Store Write : DataStoreWrite  DataStoreName=cnt_idle  IndexOptions=Index vector (dialog)  Indices=1  OutputSizes=1
  wires:
  Constant/1 -> Data Store Write/1

== system main/Task_Manager/idle/idle_task/calib ==
  note: Note:
      | calibrates one time for:
      | references
      | protection levels
      | unless change in reference during run
      | time is initiated (test purposes only)
  Action Port : ActionPort  ActionPortLabel=case [ 1 ]:
  calib : Stateflow chart  TreatAsAtomicUnit=on

== system main/Task_Manager/idle/idle_task/comm_npc ==
  Action Port : ActionPort  ActionPortLabel=case [ 4 ]:
  comm_npc : Stateflow chart  TreatAsAtomicUnit=on

== system main/Task_Manager/idle/idle_task/debug_dac ==
  Action Port : ActionPort  ActionPortLabel=case [ 5 ]:
  DAC : c2837xDlib/DAC  Commented=on  channel=B  saturate=off
      settings: SourceProductBaseCode=TIC2000
  DAC1 : c2837xDlib/DAC  Commented=on  channel=C  saturate=off
      settings: SourceProductBaseCode=TIC2000
